simulink model "pfb_fir_generic_async_test_sim4"  (R2012b)
settings: Solver=VariableStepDiscrete  StartTime=0.0  StopTime=10.0  RelTol=1e-3
model workspace (MAT data in the model file):
  synci = [0 1 2 3 4 5 6 7 8 9 10 11 ... (131074 elements, 65537x2)]
  din0 = [0 1 2 3 4 5 6 7 8 9 10 11 ... (16386 elements, 8193x2)]
  din1 = [0 1 2 3 4 5 6 7 8 9 10 11 ... (16386 elements, 8193x2)]
  din2 = [0 1 2 3 4 5 6 7 8 9 10 11 ... (16386 elements, 8193x2)]
  din3 = [0 1 2 3 4 5 6 7 8 9 10 11 ... (16386 elements, 8193x2)]
  din4 = [0 1 2 3 4 5 6 7 8 9 10 11 ... (16386 elements, 8193x2)]
  din5 = [0 1 2 3 4 5 6 7 8 9 10 11 ... (16386 elements, 8193x2)]
  din6 = [0 1 2 3 4 5 6 7 8 9 10 11 ... (16386 elements, 8193x2)]
  din7 = [0 1 2 3 4 5 6 7 8 9 10 11 ... (16386 elements, 8193x2)]
  dvalid = [0 1 2 3 4 5 6 7 8 9 10 11 ... (131072 elements, 65536x2)]
libraries: xbsIndex_r4 x3718, casper_library_delays x1
(part 8 of 18)

== system pfb_fir_generic_async_test_sim4/pfb_fir_generic/pfb_fir_coeff_gen/munge ==
  din : Inport
  join : Subsystem  AncestorBlock=casper_library_flow_control/bus_create  mask(bus_create){inputNum=32}
      mask prompts: inputNum "Number of inputs:"
      mask init:
      | bus_create_init(gcb,...
      |     'inputNum', inputNum);
  reinterpret : xbsIndex_r4/Reinterpret  force_arith_type=on  arith_type=Unsigned  force_bin_pt=on  bin_pt=0  block_type=reinterpret
  reinterpret_out : xbsIndex_r4/Reinterpret  force_arith_type=on  arith_type=Unsigned  force_bin_pt=on  bin_pt=0  block_type=reinterpret
  split : Subsystem  AncestorBlock=casper_library_flow_control/bus_expand  mask(bus_expand){mode=divisions of arbitrary size, outputNum=1, outputWidth=[18 18 18 18 18 18 18 18 18 18 18 18 18 18 18 18 18 18 18 18 18 18 18 18 18 18 18 18 18 18 18 18], outputBinaryPt=[0 0 0 0 0 0 0 0 0 0 0 0 0 0 0 0 0 0 0 0 0 0 0 0 0 0 0 0 0 0 0 0], outputArithmeticType=[0 0 0 0 0 0 0 0 0 0 0 0 0 0 0 0 0 0 0 0 0 0 0 0 0 0 0 0 0 0 0 0], show_format=off, outputToWorkspace=off, variablePrefix=out, outputToModelAsWell=on}
      mask prompts: outputNum "Number of outputs:"; outputWidth "Output width [msb ... lsb]:"; outputBinaryPt "Output binary point position [msb ... lsb]:"; outputArithmeticType "Output arithmetic type (ufix=0, fix=1, bool=2) [msb ... lsb]:"; show_format "Print format string?"; outputToWorkspace "Output to workspace?"; variablePrefix "Variable name prefix:"; outputToModelAsWell "Output to model as well?"
      mask help:
      | Expands a 'bus' made using a bus_create or Xilinx
      | concat block.
      | The input will be divided into the specified number
      | of outputs with the specified arithmetic types.
      | Divisions are made from most significant bit.
      mask init: same as pfb_fir_generic_async_test_sim4/pfb_fir_generic/bus_expand
      settings: AttributesFormatString=32 outputs
      mask TypeOptions mode: divisions of equal size | divisions of arbitrary size
      mask Callback mode: bus_expand_callback();
      mask Callback outputWidth: bus_expand_callback();
      mask Callback outputToWorkspace: bus_expand_callback();
  dout : Outport
  wires:
  reinterpret_out/1 -> dout/1
  din/1 -> reinterpret/1
  reinterpret/1 -> split/1(bus_in)
  join/1(bus_out) -> reinterpret_out/1
  split/25(out8) -> join/1(in1)
  split/32(lsb_out1) -> join/2(in2)
  split/31(out2) -> join/3(in3)
  split/30(out3) -> join/4(in4)
  split/29(out4) -> join/5(in5)
  split/28(out5) -> join/6(in6)
  split/27(out6) -> join/7(in7)
  split/26(out7) -> join/8(in8)
  split/17(out16) -> join/9(in9)
  split/24(out9) -> join/10(in10)
  split/23(out10) -> join/11(in11)
  split/22(out11) -> join/12(in12)
  split/21(out12) -> join/13(in13)
  split/20(out13) -> join/14(in14)
  split/19(out14) -> join/15(in15)
  split/18(out15) -> join/16(in16)
  split/9(out24) -> join/17(in17)
  split/16(out17) -> join/18(in18)
  split/15(out18) -> join/19(in19)
  split/14(out19) -> join/20(in20)
  split/13(out20) -> join/21(in21)
  split/12(out21) -> join/22(in22)
  split/11(out22) -> join/23(in23)
  split/10(out23) -> join/24(in24)
  split/1(msb_out32) -> join/25(in25)
  split/8(out25) -> join/26(in26)
  split/7(out26) -> join/27(in27)
  split/6(out27) -> join/28(in28)
  split/5(out28) -> join/29(in29)
  split/4(out29) -> join/30(in30)
  split/3(out30) -> join/31(in31)
  split/2(out31) -> join/32(in32)

== system pfb_fir_generic_async_test_sim4/pfb_fir_generic/pfb_fir_coeff_gen/rom ==
  addra : Inport
  dina : Inport  Port=2
  wea : Inport  Port=3
  addrb : Inport  Port=4
  dinb : Inport  Port=5
  web : Inport  Port=6
  A_bussify : Subsystem  AncestorBlock=casper_library_flow_control/bus_create  mask(bus_create){inputNum=16}
      mask prompts: inputNum "Number of inputs:"
      mask init:
      | bus_create_init(gcb,...
      |     'inputNum', inputNum);
  B_bussify : Subsystem  AncestorBlock=casper_library_flow_control/bus_create  mask(bus_create){inputNum=16}
      mask prompts: inputNum "Number of inputs:"
      mask init:
      | bus_create_init(gcb,...
      |     'inputNum', inputNum);
  bram{0..15} (16 alike) : xbsIndex_r4/Dual Port RAM  depth=1024  initVector=getfield(get_param(gcb, 'UserData'), 'initVector')  distributed_mem=Block RAM  init_a=0  init_b=0  rst_a=off  rst_b=off  en_a=off  en_b=off  latency=8  write_mode_A=Read Before Write  write_mode_B=Read Before Write  dbl_ovrd=off  optimize=Speed  block_type=dpram
  ddina : xbsIndex_r4/Delay  rst=off  infoeditControl=Selection of Reset will increase slice count due to use of real FFs and instead of SRLs  en=off  latency=0  dbl_ovrd=off  reg_retiming=on  block_type=delay
  ddinb : xbsIndex_r4/Delay  rst=off  infoeditControl=Selection of Reset will increase slice count due to use of real FFs and instead of SRLs  en=off  latency=0  dbl_ovrd=off  reg_retiming=on  block_type=delay
  debus_addra : Subsystem  AncestorBlock=casper_library_flow_control/bus_expand  mask(bus_expand){mode=divisions of equal size, outputNum=16, outputWidth=[10 10 10 10 10 10 10 10 10 10 10 10 10 10 10 10], outputBinaryPt=[0 0 0 0 0 0 0 0 0 0 0 0 0 0 0 0], outputArithmeticType=[0 0 0 0 0 0 0 0 0 0 0 0 0 0 0 0], show_format=on, outputToWorkspace=off, variablePrefix=, outputToModelAsWell=on}
      mask prompts: outputNum "Number of outputs:"; outputWidth "Output width:"; outputBinaryPt "Output binary point position:"; outputArithmeticType "Output arithmetic type (ufix=0, fix=1, bool=2):"; show_format "Print format string?"; outputToWorkspace "Output to workspace?"; variablePrefix "Variable name prefix:"; outputToModelAsWell "Output to model as well?"
      mask help:
      | Expands a 'bus' made using a bus_create or Xilinx
      | concat block.
      | The input will be divided into the specified number
      | of outputs with the specified arithmetic types.
      | Divisions are made from most significant bit.
      mask init: same as pfb_fir_generic_async_test_sim4/pfb_fir_generic/bus_expand
      settings: AttributesFormatString=16 outputs: uf10.0,uf10.0,uf10.0,uf10.0,uf10.0,uf10.0,uf10.0,uf10.0,uf10.0,uf10.0,uf10.0,uf10.0,uf10.0,uf10.0,uf10.0,uf10.0,
      mask TypeOptions mode: divisions of equal size | divisions of arbitrary size
      mask Callback mode: bus_expand_callback();
      mask Callback outputWidth: bus_expand_callback();
      mask Callback outputToWorkspace: bus_expand_callback();
  debus_addrb : Subsystem  AncestorBlock=casper_library_flow_control/bus_expand  mask(bus_expand){mode=divisions of equal size, outputNum=16, outputWidth=[10 10 10 10 10 10 10 10 10 10 10 10 10 10 10 10], outputBinaryPt=[0 0 0 0 0 0 0 0 0 0 0 0 0 0 0 0], outputArithmeticType=[0 0 0 0 0 0 0 0 0 0 0 0 0 0 0 0], show_format=on, outputToWorkspace=off, variablePrefix=, outputToModelAsWell=on}
      mask prompts: outputNum "Number of outputs:"; outputWidth "Output width:"; outputBinaryPt "Output binary point position:"; outputArithmeticType "Output arithmetic type (ufix=0, fix=1, bool=2):"; show_format "Print format string?"; outputToWorkspace "Output to workspace?"; variablePrefix "Variable name prefix:"; outputToModelAsWell "Output to model as well?"
      mask help:
      | Expands a 'bus' made using a bus_create or Xilinx
      | concat block.
      | The input will be divided into the specified number
      | of outputs with the specified arithmetic types.
      | Divisions are made from most significant bit.
      mask init: same as pfb_fir_generic_async_test_sim4/pfb_fir_generic/bus_expand
      settings: AttributesFormatString=16 outputs: uf10.0,uf10.0,uf10.0,uf10.0,uf10.0,uf10.0,uf10.0,uf10.0,uf10.0,uf10.0,uf10.0,uf10.0,uf10.0,uf10.0,uf10.0,uf10.0,
      mask TypeOptions mode: divisions of equal size | divisions of arbitrary size
      mask Callback mode: bus_expand_callback();
      mask Callback outputWidth: bus_expand_callback();
      mask Callback outputToWorkspace: bus_expand_callback();
  debus_dina : Subsystem  AncestorBlock=casper_library_flow_control/bus_expand  mask(bus_expand){mode=divisions of arbitrary size, outputNum=1, outputWidth=[36 36 36 36 36 36 36 36 36 36 36 36 36 36 36 36], outputBinaryPt=[0 0 0 0 0 0 0 0 0 0 0 0 0 0 0 0], outputArithmeticType=[0 0 0 0 0 0 0 0 0 0 0 0 0 0 0 0], show_format=on, outputToWorkspace=off, variablePrefix=, outputToModelAsWell=on}
      mask prompts: outputNum "Number of outputs:"; outputWidth "Output width [msb ... lsb]:"; outputBinaryPt "Output binary point position [msb ... lsb]:"; outputArithmeticType "Output arithmetic type (ufix=0, fix=1, bool=2) [msb ... lsb]:"; show_format "Print format string?"; outputToWorkspace "Output to workspace?"; variablePrefix "Variable name prefix:"; outputToModelAsWell "Output to model as well?"
      mask help:
      | Expands a 'bus' made using a bus_create or Xilinx
      | concat block.
      | The input will be divided into the specified number
      | of outputs with the specified arithmetic types.
      | Divisions are made from most significant bit.
      mask init: same as pfb_fir_generic_async_test_sim4/pfb_fir_generic/bus_expand
      settings: AttributesFormatString=16 outputs: uf36.0,uf36.0,uf36.0,uf36.0,uf36.0,uf36.0,uf36.0,uf36.0,uf36.0,uf36.0,uf36.0,uf36.0,uf36.0,uf36.0,uf36.0,uf36.0,
      mask TypeOptions mode: divisions of equal size | divisions of arbitrary size
      mask Callback mode: bus_expand_callback();
      mask Callback outputWidth: bus_expand_callback();
      mask Callback outputToWorkspace: bus_expand_callback();
  debus_dinb : Subsystem  AncestorBlock=casper_library_flow_control/bus_expand  mask(bus_expand){mode=divisions of arbitrary size, outputNum=1, outputWidth=[36 36 36 36 36 36 36 36 36 36 36 36 36 36 36 36], outputBinaryPt=[0 0 0 0 0 0 0 0 0 0 0 0 0 0 0 0], outputArithmeticType=[0 0 0 0 0 0 0 0 0 0 0 0 0 0 0 0], show_format=on, outputToWorkspace=off, variablePrefix=, outputToModelAsWell=on}
      mask prompts: outputNum "Number of outputs:"; outputWidth "Output width [msb ... lsb]:"; outputBinaryPt "Output binary point position [msb ... lsb]:"; outputArithmeticType "Output arithmetic type (ufix=0, fix=1, bool=2) [msb ... lsb]:"; show_format "Print format string?"; outputToWorkspace "Output to workspace?"; variablePrefix "Variable name prefix:"; outputToModelAsWell "Output to model as well?"
      mask help:
      | Expands a 'bus' made using a bus_create or Xilinx
      | concat block.
      | The input will be divided into the specified number
      | of outputs with the specified arithmetic types.
      | Divisions are made from most significant bit.
      mask init: same as pfb_fir_generic_async_test_sim4/pfb_fir_generic/bus_expand
      settings: AttributesFormatString=16 outputs: uf36.0,uf36.0,uf36.0,uf36.0,uf36.0,uf36.0,uf36.0,uf36.0,uf36.0,uf36.0,uf36.0,uf36.0,uf36.0,uf36.0,uf36.0,uf36.0,
      mask TypeOptions mode: divisions of equal size | divisions of arbitrary size
      mask Callback mode: bus_expand_callback();
      mask Callback outputWidth: bus_expand_callback();
      mask Callback outputToWorkspace: bus_expand_callback();
  debus_wea : Subsystem  AncestorBlock=casper_library_flow_control/bus_expand  mask(bus_expand){mode=divisions of equal size, outputNum=16, outputWidth=[1 1 1 1 1 1 1 1 1 1 1 1 1 1 1 1], outputBinaryPt=[0 0 0 0 0 0 0 0 0 0 0 0 0 0 0 0], outputArithmeticType=[2 2 2 2 2 2 2 2 2 2 2 2 2 2 2 2], show_format=on, outputToWorkspace=off, variablePrefix=, outputToModelAsWell=on}
      mask prompts: outputNum "Number of outputs:"; outputWidth "Output width:"; outputBinaryPt "Output binary point position:"; outputArithmeticType "Output arithmetic type (ufix=0, fix=1, bool=2):"; show_format "Print format string?"; outputToWorkspace "Output to workspace?"; variablePrefix "Variable name prefix:"; outputToModelAsWell "Output to model as well?"
      mask help:
      | Expands a 'bus' made using a bus_create or Xilinx
      | concat block.
      | The input will be divided into the specified number
      | of outputs with the specified arithmetic types.
      | Divisions are made from most significant bit.
      mask init: same as pfb_fir_generic_async_test_sim4/pfb_fir_generic/bus_expand
      settings: AttributesFormatString=16 outputs: b,b,b,b,b,b,b,b,b,b,b,b,b,b,b,b,
      mask TypeOptions mode: divisions of equal size | divisions of arbitrary size
      mask Callback mode: bus_expand_callback();
      mask Callback outputWidth: bus_expand_callback();
      mask Callback outputToWorkspace: bus_expand_callback();
  debus_web : Subsystem  AncestorBlock=casper_library_flow_control/bus_expand  mask(bus_expand){mode=divisions of equal size, outputNum=16, outputWidth=[1 1 1 1 1 1 1 1 1 1 1 1 1 1 1 1], outputBinaryPt=[0 0 0 0 0 0 0 0 0 0 0 0 0 0 0 0], outputArithmeticType=[2 2 2 2 2 2 2 2 2 2 2 2 2 2 2 2], show_format=on, outputToWorkspace=off, variablePrefix=, outputToModelAsWell=on}
      mask prompts: outputNum "Number of outputs:"; outputWidth "Output width:"; outputBinaryPt "Output binary point position:"; outputArithmeticType "Output arithmetic type (ufix=0, fix=1, bool=2):"; show_format "Print format string?"; outputToWorkspace "Output to workspace?"; variablePrefix "Variable name prefix:"; outputToModelAsWell "Output to model as well?"
      mask help:
      | Expands a 'bus' made using a bus_create or Xilinx
      | concat block.
      | The input will be divided into the specified number
      | of outputs with the specified arithmetic types.
      | Divisions are made from most significant bit.
      mask init: same as pfb_fir_generic_async_test_sim4/pfb_fir_generic/bus_expand
      settings: AttributesFormatString=16 outputs: b,b,b,b,b,b,b,b,b,b,b,b,b,b,b,b,
      mask TypeOptions mode: divisions of equal size | divisions of arbitrary size
      mask Callback mode: bus_expand_callback();
      mask Callback outputWidth: bus_expand_callback();
      mask Callback outputToWorkspace: bus_expand_callback();
  rep_addra : Subsystem  AncestorBlock=casper_library_bus/bus_replicate  mask(bus_replicate){replication=16, latency=9, misc=off, implementation=core}
      mask prompts: replication "replication factor"; misc "misc support"; implementation "delay implementation"
      mask help: Output bus formed by replicating input bus a number of times
      mask init:
      | bus_replicate_init(gcb, ...
      |     'replication', replication, ...
      |     'latency', latency, ...
      |     'implementation', implementation, ...
      |     'misc', misc);
      mask TypeOptions implementation: core | behavioral
  rep_addrb : Subsystem  AncestorBlock=casper_library_bus/bus_replicate  mask(bus_replicate){replication=16, latency=9, misc=off, implementation=core}
      mask prompts: replication "replication factor"; misc "misc support"; implementation "delay implementation"
      mask help: Output bus formed by replicating input bus a number of times
      mask init:
      | bus_replicate_init(gcb, ...
      |     'replication', replication, ...
      |     'latency', latency, ...
      |     'implementation', implementation, ...
      |     'misc', misc);
      mask TypeOptions implementation: core | behavioral
  rep_wea : Subsystem  AncestorBlock=casper_library_bus/bus_replicate  mask(bus_replicate){replication=16, latency=0, misc=off, implementation=behavioral}
      mask prompts: replication "replication factor"; misc "misc support"; implementation "delay implementation"
      mask help: Output bus formed by replicating input bus a number of times
      mask init:
      | bus_replicate_init(gcb, ...
      |     'replication', replication, ...
      |     'latency', latency, ...
      |     'implementation', implementation, ...
      |     'misc', misc);
      mask TypeOptions implementation: core | behavioral
  rep_web : Subsystem  AncestorBlock=casper_library_bus/bus_replicate  mask(bus_replicate){replication=16, latency=0, misc=off, implementation=behavioral}
      mask prompts: replication "replication factor"; misc "misc support"; implementation "delay implementation"
      mask help: Output bus formed by replicating input bus a number of times
      mask init:
      | bus_replicate_init(gcb, ...
      |     'replication', replication, ...
      |     'latency', latency, ...
      |     'implementation', implementation, ...
      |     'misc', misc);
      mask TypeOptions implementation: core | behavioral
  A : Outport
  B : Outport  Port=2
  wires:
  addra/1 -> rep_addra/1(in)
  dina/1 -> ddina/1
  wea/1 -> rep_wea/1(in)
  addrb/1 -> rep_addrb/1(in)
  dinb/1 -> ddinb/1
  web/1 -> rep_web/1(in)
  rep_addra/1(out) -> debus_addra/1(bus_in)
  ddina/1 -> debus_dina/1(bus_in)
  rep_wea/1(out) -> debus_wea/1(bus_in)
  rep_addrb/1(out) -> debus_addrb/1(bus_in)
  ddinb/1 -> debus_dinb/1(bus_in)
  rep_web/1(out) -> debus_web/1(bus_in)
  debus_addra/1(msb_out16) -> bram0/1
  debus_dina/1(msb_out16) -> bram0/2
  debus_wea/1(msb_out16) -> bram0/3
  debus_addrb/1(msb_out16) -> bram0/4
  debus_dinb/1(msb_out16) -> bram0/5
  debus_web/1(msb_out16) -> bram0/6
  debus_addra/2(out15) -> bram1/1
  debus_dina/2(out15) -> bram1/2
  debus_wea/2(out15) -> bram1/3
  debus_addrb/2(out15) -> bram1/4
  debus_dinb/2(out15) -> bram1/5
  debus_web/2(out15) -> bram1/6
  debus_addra/3(out14) -> bram2/1
  debus_dina/3(out14) -> bram2/2
  debus_wea/3(out14) -> bram2/3
  debus_addrb/3(out14) -> bram2/4
  debus_dinb/3(out14) -> bram2/5
  debus_web/3(out14) -> bram2/6
  debus_addra/4(out13) -> bram3/1
  debus_dina/4(out13) -> bram3/2
  debus_wea/4(out13) -> bram3/3
  debus_addrb/4(out13) -> bram3/4
  debus_dinb/4(out13) -> bram3/5
  debus_web/4(out13) -> bram3/6
  debus_addra/5(out12) -> bram4/1
  debus_dina/5(out12) -> bram4/2
  debus_wea/5(out12) -> bram4/3
  debus_addrb/5(out12) -> bram4/4
  debus_dinb/5(out12) -> bram4/5
  debus_web/5(out12) -> bram4/6
  debus_addra/6(out11) -> bram5/1
  debus_dina/6(out11) -> bram5/2
  debus_wea/6(out11) -> bram5/3
  debus_addrb/6(out11) -> bram5/4
  debus_dinb/6(out11) -> bram5/5
  debus_web/6(out11) -> bram5/6
  debus_addra/7(out10) -> bram6/1
  debus_dina/7(out10) -> bram6/2
  debus_wea/7(out10) -> bram6/3
  debus_addrb/7(out10) -> bram6/4
  debus_dinb/7(out10) -> bram6/5
  debus_web/7(out10) -> bram6/6
  debus_addra/8(out9) -> bram7/1
  debus_dina/8(out9) -> bram7/2
  debus_wea/8(out9) -> bram7/3
  debus_addrb/8(out9) -> bram7/4
  debus_dinb/8(out9) -> bram7/5
  debus_web/8(out9) -> bram7/6
  debus_addra/9(out8) -> bram8/1
  debus_dina/9(out8) -> bram8/2
  debus_wea/9(out8) -> bram8/3
  debus_addrb/9(out8) -> bram8/4
  debus_dinb/9(out8) -> bram8/5
  debus_web/9(out8) -> bram8/6
  debus_addra/10(out7) -> bram9/1
  debus_dina/10(out7) -> bram9/2
  debus_wea/10(out7) -> bram9/3
  debus_addrb/10(out7) -> bram9/4
  debus_dinb/10(out7) -> bram9/5
  debus_web/10(out7) -> bram9/6
  debus_addra/11(out6) -> bram10/1
  debus_dina/11(out6) -> bram10/2
  debus_wea/11(out6) -> bram10/3
  debus_addrb/11(out6) -> bram10/4
  debus_dinb/11(out6) -> bram10/5
  debus_web/11(out6) -> bram10/6
  debus_addra/12(out5) -> bram11/1
  debus_dina/12(out5) -> bram11/2
  debus_wea/12(out5) -> bram11/3
  debus_addrb/12(out5) -> bram11/4
  debus_dinb/12(out5) -> bram11/5
  debus_web/12(out5) -> bram11/6
  debus_addra/13(out4) -> bram12/1
  debus_dina/13(out4) -> bram12/2
  debus_wea/13(out4) -> bram12/3
  debus_addrb/13(out4) -> bram12/4
  debus_dinb/13(out4) -> bram12/5
  debus_web/13(out4) -> bram12/6
  debus_addra/14(out3) -> bram13/1
  debus_dina/14(out3) -> bram13/2
  debus_wea/14(out3) -> bram13/3
  debus_addrb/14(out3) -> bram13/4
  debus_dinb/14(out3) -> bram13/5
  debus_web/14(out3) -> bram13/6
  debus_addra/15(out2) -> bram14/1
  debus_dina/15(out2) -> bram14/2
  debus_wea/15(out2) -> bram14/3
  debus_addrb/15(out2) -> bram14/4
  debus_dinb/15(out2) -> bram14/5
  debus_web/15(out2) -> bram14/6
  debus_addra/16(lsb_out1) -> bram15/1
  debus_dina/16(lsb_out1) -> bram15/2
  debus_wea/16(lsb_out1) -> bram15/3
  debus_addrb/16(lsb_out1) -> bram15/4
  debus_dinb/16(lsb_out1) -> bram15/5
  debus_web/16(lsb_out1) -> bram15/6
  bram0/1 -> A_bussify/1(in1)
  bram0/2 -> B_bussify/1(in1)
  bram1/1 -> A_bussify/2(in2)
  bram1/2 -> B_bussify/2(in2)
  bram2/1 -> A_bussify/3(in3)
  bram2/2 -> B_bussify/3(in3)
  bram3/1 -> A_bussify/4(in4)
  bram3/2 -> B_bussify/4(in4)
  bram4/1 -> A_bussify/5(in5)
  bram4/2 -> B_bussify/5(in5)
  bram5/1 -> A_bussify/6(in6)
  bram5/2 -> B_bussify/6(in6)
  bram6/1 -> A_bussify/7(in7)
  bram6/2 -> B_bussify/7(in7)
  bram7/1 -> A_bussify/8(in8)
  bram7/2 -> B_bussify/8(in8)
  bram8/1 -> A_bussify/9(in9)
  bram8/2 -> B_bussify/9(in9)
  bram9/1 -> A_bussify/10(in10)
  bram9/2 -> B_bussify/10(in10)
  bram10/1 -> A_bussify/11(in11)
  bram10/2 -> B_bussify/11(in11)
  bram11/1 -> A_bussify/12(in12)
  bram11/2 -> B_bussify/12(in12)
  bram12/1 -> A_bussify/13(in13)
  bram12/2 -> B_bussify/13(in13)
  bram13/1 -> A_bussify/14(in14)
  bram13/2 -> B_bussify/14(in14)
  bram14/1 -> A_bussify/15(in15)
  bram14/2 -> B_bussify/15(in15)
  bram15/1 -> A_bussify/16(in16)
  bram15/2 -> B_bussify/16(in16)
  A_bussify/1(bus_out) -> A/1
  B_bussify/1(bus_out) -> B/1
